simulink model "gg_plus_lc_platoon"  (R2019a)
settings: Solver=ode23t  StartTime=0.0  StopTime=70  FixedStep=0.1  MaxStep=0.01  RelTol=1e-3
InitFcn:
  | load vehStatesBus
libraries: simulink x120, powerlib_meascontrol x14, dspsigops x7, autolibshared x7
(part 2 of 7)

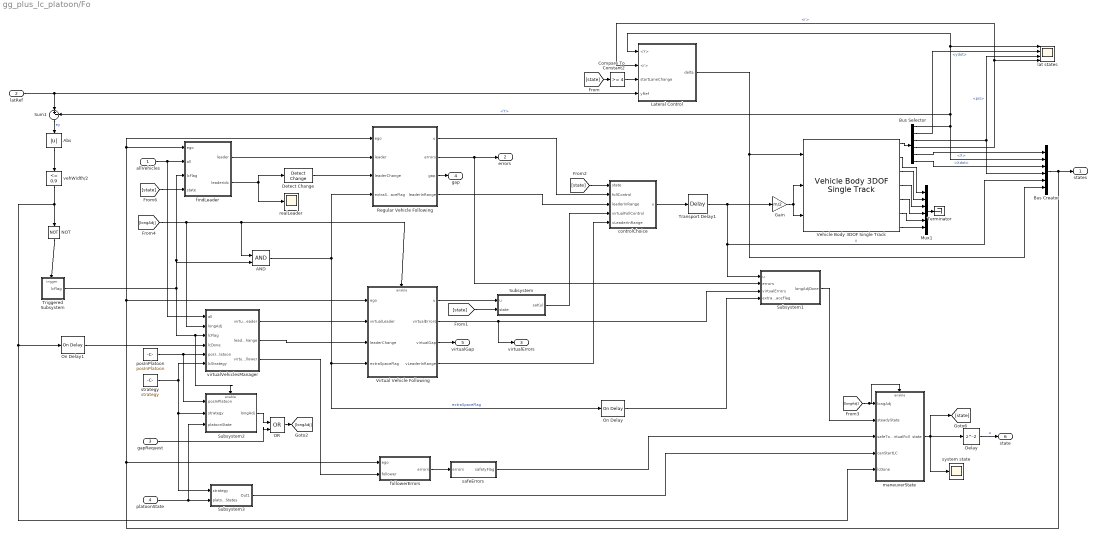
== system gg_plus_lc_platoon/Fo ==
  allVehicles : Inport
  latRef : Inport  Port=2
  gapRequest : Inport  Port=3
  platoonState : Inport  Port=4
  AND : Logic  IconShape=distinctive  AllPortsSameDT=off  OutDataTypeStr=boolean
  Abs : Abs
  Bus Creator : BusCreator  Inputs=6  OutDataTypeStr=Bus: vehStatesBus  NonVirtualBus=on
  Bus Selector : BusSelector  OutputSignals=InertFrm.Cg.Disp.Y,BdyFrm.Cg.Vel.ydot,InertFrm.Cg.Ang.psi,BdyFrm.Cg.AngVel.r,InertFrm.RearAxl.Disp.X,InertFrm.RearAxl.Vel.Xdot
  Compare To Constant2 : simulink/Logic and Bit Operations/Compare To Constant  relop=>=  const=4  OutDataTypeStr=boolean
  Delay : Delay
  Detect Change : simulink/Logic and Bit Operations/Detect Change  vinit=0  OutDataTypeStr=boolean
  Gain : Gain  Gain=m/2
  Lateral Control : Subsystem
  Mux1 : Mux  Inputs=6
  NOT : Logic  Operator=NOT  IconShape=distinctive  AllPortsSameDT=off  OutDataTypeStr=boolean
  OR : Logic  Operator=OR  IconShape=distinctive  AllPortsSameDT=off  OutDataTypeStr=boolean
  On Delay : powerlib_meascontrol/Logic/On Delay  DelayType=On delay  delay=1  ic=0  Ts=0
      settings: SourceProductName=Simscape Electrical
  On Delay1 : powerlib_meascontrol/Logic/On Delay  DelayType=On delay  delay=0.1  ic=0  Ts=0
      settings: SourceProductName=Simscape Electrical
  Regular Vehicle Following : Subsystem
  Subsystem : Subsystem
  Subsystem1 : Subsystem
  Subsystem2 : Subsystem
  Subsystem3 : Subsystem
  Sum1 : Sum  Inputs=|+-
  Terminator : Terminator
  Transport Delay1 : TransportDelay  DelayTime=0.01
  Triggered Subsystem : Subsystem  TreatAsAtomicUnit=on
  Vehicle Body 3DOF Single Track : autolibshared/Vehicle Body 3DOF Single Track  trackMode=Single (bicycle)  inputMode=External longitudinal forces  frontSteerMode=on  rearSteerMode=off  windMode=off  muMode=off  extFMode=off  extMMode=off  extXo=off  extpsio=off  extxdoto=off  extro=off  extYo=off  extTamb=off  extydoto=off  aMode=2  NF=2  NR=2  m=m  a=lf  b=lr  h=0.35  X_o=x0  xdot_o=vx0  CalphaMode=off  sigmaMode=on  d=0  w=[1.4,1.4]  Cy_f=12e3  Cy_r=11e3  sigma_f=.1  sigma_r=.1  alpha_f_brk=[-.1 .1]  Cy_f_data=[-9e3 9e3]  alpha_r_brk=[-.1 .1]  Cy_r_data=[-9e3 9e3]  Y_o=y0  ydot_o=0  Izz=4000  psi_o=0  r_o=0  Af=2  Cd=.3  Cl=.1  Cpm=.1  beta_w=[0:0.01:0.3]  Cs=[0:0.03:0.9]  Cym=[0:0.01:0.3]  Pabs=101325  Tair=273  g=9.81  mu=1  xdot_tol=.01  Fznom=5000  Fxtire_sat=7e4  Fytire_sat=7e4  longOff=0  latOff=0  vertOff=0  wrapAng=off
      settings: SourceProductName=Powertrain Blockset  SourceProductBaseCode=PW
  Virtual Vehicle Following : Subsystem  TreatAsAtomicUnit=on
  controlChoice : Subsystem
  findLeader : Subsystem
  followerErrors : Subsystem
  lat states : Scope  NumInputPorts=4
  maneuverState : Subsystem
  posInPlatoon : Constant  Value=posInPlatoon
  realLeader : Scope
  safeErrors : Subsystem
  strategy : Constant  Value=strategy
  system state : Scope
  vehWidth/2 : simulink/Logic and Bit Operations/Compare To Constant  relop=<=  const=0.9  OutDataTypeStr=boolean
  virtualVehiclesManager : Subsystem  TreatAsAtomicUnit=on
  states : Outport
  errors : Outport  Port=2
  virtualErrors : Outport  Port=3
  gap : Outport  Port=4
  virtualGap : Outport  Port=5
  state : Outport  Port=6
  wires:
  Triggered Subsystem/1(lcFlag) -> Subsystem2/Enable, virtualVehiclesManager/3(lcFlag), findLeader/3(lcFlag), AND/2
  Virtual Vehicle Following/4(vLeaderInRange) -> controlChoice/5(vLeaderInRange)
  [state] -> findLeader/4(state)
  Subsystem3/1(Out1) -> maneuverState/4(canStartLC)
  strategy/1 -> virtualVehiclesManager/6(lcStrategy), Subsystem3/1(strategy), Subsystem2/2(strategy)
  Delay/1 -> state/1  "u"
  Subsystem2/1(longAdj) -> OR/1
  platoonState/1 -> Subsystem2/3(platoonState), Subsystem3/2(platoonStates)
  [state] -> Compare To Constant2/1
  Virtual Vehicle Following/3(virtualGap) -> virtualGap/1
  maneuverState/1(state) -> Delay/1, [state], system state/1
  Lateral Control/1(delta) -> Bus Creator/6, Vehicle Body 3DOF Single Track/1
  Compare To Constant2/1 -> Lateral Control/3(startLaneChange)
  Regular Vehicle Following/2(errors) -> errors/1, Subsystem1/2(errors)
  Virtual Vehicle Following/1(u) -> Subsystem/1(u)
  Regular Vehicle Following/1(u) -> controlChoice/2(follControl)
  Regular Vehicle Following/3(gap) -> gap/1
  followerErrors/1(errors) -> safeErrors/1(errors)
  allVehicles/1 -> virtualVehiclesManager/1(all), findLeader/2(all)
  Abs/1 -> vehWidth/2/1
  AND/1 -> Regular Vehicle Following/4(extraSpaceFlag), On Delay/1, Virtual Vehicle Following/4(extraSpaceFlag)  "extraSpaceFlag"
  Bus Selector/6 -> Bus Creator/3  "<Xdot>"
  Bus Selector/5 -> Bus Creator/1  "<X>"
  Gain/1 -> Vehicle Body 3DOF Single Track/2, Vehicle Body 3DOF Single Track/3
  Vehicle Body 3DOF Single Track/1 -> Bus Selector/1
  Vehicle Body 3DOF Single Track/4 -> Mux1/3
  Vehicle Body 3DOF Single Track/3 -> Mux1/2
  Vehicle Body 3DOF Single Track/2 -> Mux1/1
  Vehicle Body 3DOF Single Track/5 -> Mux1/4
  Vehicle Body 3DOF Single Track/6 -> Mux1/5
  Vehicle Body 3DOF Single Track/7 -> Mux1/6
  Mux1/1 -> Terminator/1
  Bus Selector/1 -> Bus Creator/2, lat states/1, Lateral Control/1(<Y>), Sum1/2  "<Y>"
  Bus Selector/2 -> lat states/2  "<ydot>"
  Bus Selector/3 -> Bus Creator/4, lat states/3  "<psi>"
  Bus Selector/4 -> lat states/4, Lateral Control/2(<r>)  "<r>"
  latRef/1 -> Sum1/1, Lateral Control/4(yRef)
  Bus Creator/1 -> Regular Vehicle Following/1(ego), findLeader/1(ego), Virtual Vehicle Following/1(ego), followerErrors/1(ego), states/1
  Transport Delay1/1 -> Gain/1, Subsystem1/1(u), Bus Creator/5  "u"
  Sum1/1 -> Abs/1  "ey"
  Virtual Vehicle Following/2(virtualErrors) -> virtualErrors/1, Subsystem1/3(virtualErrors)
  Detect Change/1 -> Regular Vehicle Following/3(leaderChange)
  Subsystem/1(sat(u)) -> controlChoice/4(virtualFollControl)
  Regular Vehicle Following/4(leaderInRange) -> controlChoice/3(leaderInRange)
  findLeader/1(leader) -> Regular Vehicle Following/2(leader)
  findLeader/2(leaderIdx) -> Detect Change/1, realLeader/1
  On Delay/1 -> Subsystem1/4(extraSpaceFlag)
  NOT/1 -> Triggered Subsystem/Trigger
  [state] -> Subsystem/2(state)
  posInPlatoon/1 -> virtualVehiclesManager/5(posInPlatoon), Subsystem2/1(posInPlatoon)
  virtualVehiclesManager/1(virtualLeader) -> Virtual Vehicle Following/2(virtualLeader)
  virtualVehiclesManager/3(virtualFollower) -> followerErrors/2(follower)
  [longAdj] -> maneuverState/Enable, maneuverState/1(longAdj)
  Subsystem1/1(longAdjDone) -> maneuverState/2(steadyState)
  safeErrors/1(safetyFlag) -> maneuverState/3(safeToVirtualFoll)
  vehWidth/2/1 -> On Delay1/1, maneuverState/5(lcDone), NOT/1
  [state] -> controlChoice/1(state)
  controlChoice/1(u) -> Transport Delay1/1
  [longAdj] -> virtualVehiclesManager/2(longAdj), AND/1, Virtual Vehicle Following/Enable
  On Delay1/1 -> virtualVehiclesManager/4(lcDone)
  virtualVehiclesManager/2(leaderChange) -> Virtual Vehicle Following/3(leaderChange)
  OR/1 -> [longAdj]
  gapRequest/1 -> OR/2

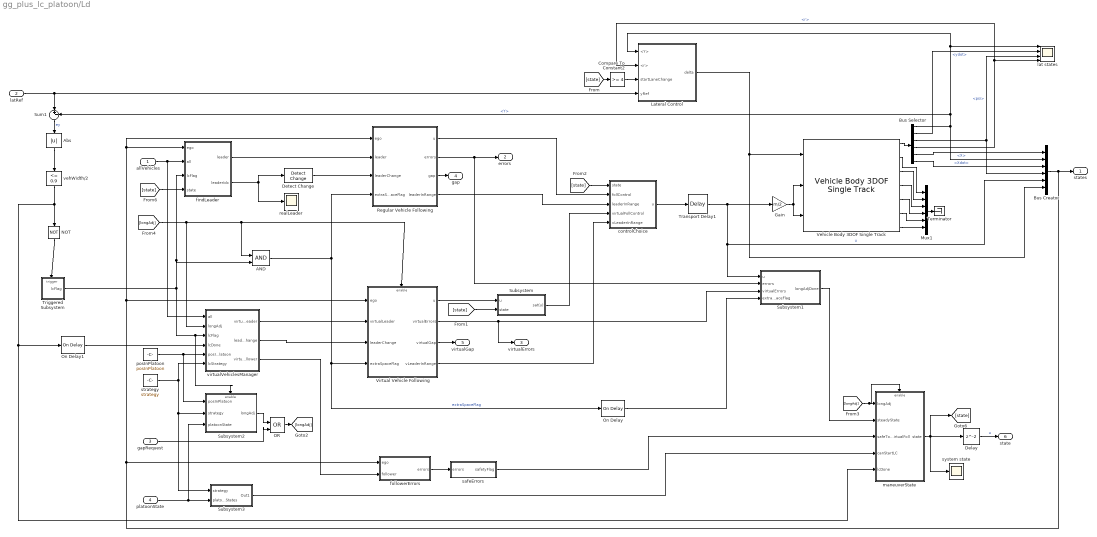
== system gg_plus_lc_platoon/Ld ==
  allVehicles : Inport
  latRef : Inport  Port=2
  gapRequest : Inport  Port=3
  platoonState : Inport  Port=4
  AND : Logic  IconShape=distinctive  AllPortsSameDT=off  OutDataTypeStr=boolean
  Abs : Abs
  Bus Creator : BusCreator  Inputs=6  OutDataTypeStr=Bus: vehStatesBus  NonVirtualBus=on
  Bus Selector : BusSelector  OutputSignals=InertFrm.Cg.Disp.Y,BdyFrm.Cg.Vel.ydot,InertFrm.Cg.Ang.psi,BdyFrm.Cg.AngVel.r,InertFrm.RearAxl.Disp.X,InertFrm.RearAxl.Vel.Xdot
  Compare To Constant2 : simulink/Logic and Bit Operations/Compare To Constant  relop=>=  const=4  OutDataTypeStr=boolean
  Delay : Delay
  Detect Change : simulink/Logic and Bit Operations/Detect Change  vinit=0  OutDataTypeStr=boolean
  Gain : Gain  Gain=m/2
  Lateral Control : Subsystem
  Mux1 : Mux  Inputs=6
  NOT : Logic  Operator=NOT  IconShape=distinctive  AllPortsSameDT=off  OutDataTypeStr=boolean
  OR : Logic  Operator=OR  IconShape=distinctive  AllPortsSameDT=off  OutDataTypeStr=boolean
  On Delay : powerlib_meascontrol/Logic/On Delay  DelayType=On delay  delay=1  ic=0  Ts=0
      settings: SourceProductName=Simscape Electrical
  On Delay1 : powerlib_meascontrol/Logic/On Delay  DelayType=On delay  delay=0.1  ic=0  Ts=0
      settings: SourceProductName=Simscape Electrical
  Regular Vehicle Following : Subsystem
  Subsystem : Subsystem
  Subsystem1 : Subsystem
  Subsystem2 : Subsystem
  Subsystem3 : Subsystem
  Sum1 : Sum  Inputs=|+-
  Terminator : Terminator
  Transport Delay1 : TransportDelay  DelayTime=0.01
  Triggered Subsystem : Subsystem  TreatAsAtomicUnit=on
  Vehicle Body 3DOF Single Track : autolibshared/Vehicle Body 3DOF Single Track  trackMode=Single (bicycle)  inputMode=External longitudinal forces  frontSteerMode=on  rearSteerMode=off  windMode=off  muMode=off  extFMode=off  extMMode=off  extXo=off  extpsio=off  extxdoto=off  extro=off  extYo=off  extTamb=off  extydoto=off  aMode=2  NF=2  NR=2  m=m  a=lf  b=lr  h=0.35  X_o=x0  xdot_o=vx0  CalphaMode=off  sigmaMode=on  d=0  w=[1.4,1.4]  Cy_f=12e3  Cy_r=11e3  sigma_f=.1  sigma_r=.1  alpha_f_brk=[-.1 .1]  Cy_f_data=[-9e3 9e3]  alpha_r_brk=[-.1 .1]  Cy_r_data=[-9e3 9e3]  Y_o=y0  ydot_o=0  Izz=4000  psi_o=0  r_o=0  Af=2  Cd=.3  Cl=.1  Cpm=.1  beta_w=[0:0.01:0.3]  Cs=[0:0.03:0.9]  Cym=[0:0.01:0.3]  Pabs=101325  Tair=273  g=9.81  mu=1  xdot_tol=.01  Fznom=5000  Fxtire_sat=7e4  Fytire_sat=7e4  longOff=0  latOff=0  vertOff=0  wrapAng=off
      settings: SourceProductName=Powertrain Blockset  SourceProductBaseCode=PW
  Virtual Vehicle Following : Subsystem  TreatAsAtomicUnit=on
  controlChoice : Subsystem
  findLeader : Subsystem
  followerErrors : Subsystem
  lat states : Scope  NumInputPorts=4
  maneuverState : Subsystem
  posInPlatoon : Constant  Value=posInPlatoon
  realLeader : Scope
  safeErrors : Subsystem
  strategy : Constant  Value=strategy
  system state : Scope
  vehWidth/2 : simulink/Logic and Bit Operations/Compare To Constant  relop=<=  const=0.9  OutDataTypeStr=boolean
  virtualVehiclesManager : Subsystem  TreatAsAtomicUnit=on
  states : Outport
  errors : Outport  Port=2
  virtualErrors : Outport  Port=3
  gap : Outport  Port=4
  virtualGap : Outport  Port=5
  state : Outport  Port=6
  wires:
  Triggered Subsystem/1(lcFlag) -> Subsystem2/Enable, virtualVehiclesManager/3(lcFlag), findLeader/3(lcFlag), AND/2
  Virtual Vehicle Following/4(vLeaderInRange) -> controlChoice/5(vLeaderInRange)
  [state] -> findLeader/4(state)
  Subsystem3/1(Out1) -> maneuverState/4(canStartLC)
  strategy/1 -> virtualVehiclesManager/6(lcStrategy), Subsystem3/1(strategy), Subsystem2/2(strategy)
  Delay/1 -> state/1  "u"
  Subsystem2/1(longAdj) -> OR/1
  platoonState/1 -> Subsystem2/3(platoonState), Subsystem3/2(platoonStates)
  [state] -> Compare To Constant2/1
  Virtual Vehicle Following/3(virtualGap) -> virtualGap/1
  maneuverState/1(state) -> Delay/1, [state], system state/1
  Lateral Control/1(delta) -> Bus Creator/6, Vehicle Body 3DOF Single Track/1
  Compare To Constant2/1 -> Lateral Control/3(startLaneChange)
  Regular Vehicle Following/2(errors) -> errors/1, Subsystem1/2(errors)
  Virtual Vehicle Following/1(u) -> Subsystem/1(u)
  Regular Vehicle Following/1(u) -> controlChoice/2(follControl)
  Regular Vehicle Following/3(gap) -> gap/1
  followerErrors/1(errors) -> safeErrors/1(errors)
  allVehicles/1 -> virtualVehiclesManager/1(all), findLeader/2(all)
  Abs/1 -> vehWidth/2/1
  AND/1 -> Regular Vehicle Following/4(extraSpaceFlag), On Delay/1, Virtual Vehicle Following/4(extraSpaceFlag)  "extraSpaceFlag"
  Bus Selector/6 -> Bus Creator/3  "<Xdot>"
  Bus Selector/5 -> Bus Creator/1  "<X>"
  Gain/1 -> Vehicle Body 3DOF Single Track/2, Vehicle Body 3DOF Single Track/3
  Vehicle Body 3DOF Single Track/1 -> Bus Selector/1
  Vehicle Body 3DOF Single Track/4 -> Mux1/3
  Vehicle Body 3DOF Single Track/3 -> Mux1/2
  Vehicle Body 3DOF Single Track/2 -> Mux1/1
  Vehicle Body 3DOF Single Track/5 -> Mux1/4
  Vehicle Body 3DOF Single Track/6 -> Mux1/5
  Vehicle Body 3DOF Single Track/7 -> Mux1/6
  Mux1/1 -> Terminator/1
  Bus Selector/1 -> Bus Creator/2, lat states/1, Lateral Control/1(<Y>), Sum1/2  "<Y>"
  Bus Selector/2 -> lat states/2  "<ydot>"
  Bus Selector/3 -> Bus Creator/4, lat states/3  "<psi>"
  Bus Selector/4 -> lat states/4, Lateral Control/2(<r>)  "<r>"
  latRef/1 -> Sum1/1, Lateral Control/4(yRef)
  Bus Creator/1 -> Regular Vehicle Following/1(ego), findLeader/1(ego), Virtual Vehicle Following/1(ego), followerErrors/1(ego), states/1
  Transport Delay1/1 -> Gain/1, Subsystem1/1(u), Bus Creator/5  "u"
  Sum1/1 -> Abs/1  "ey"
  Virtual Vehicle Following/2(virtualErrors) -> virtualErrors/1, Subsystem1/3(virtualErrors)
  Detect Change/1 -> Regular Vehicle Following/3(leaderChange)
  Subsystem/1(sat(u)) -> controlChoice/4(virtualFollControl)
  Regular Vehicle Following/4(leaderInRange) -> controlChoice/3(leaderInRange)
  findLeader/1(leader) -> Regular Vehicle Following/2(leader)
  findLeader/2(leaderIdx) -> Detect Change/1, realLeader/1
  On Delay/1 -> Subsystem1/4(extraSpaceFlag)
  NOT/1 -> Triggered Subsystem/Trigger
  [state] -> Subsystem/2(state)
  posInPlatoon/1 -> virtualVehiclesManager/5(posInPlatoon), Subsystem2/1(posInPlatoon)
  virtualVehiclesManager/1(virtualLeader) -> Virtual Vehicle Following/2(virtualLeader)
  virtualVehiclesManager/3(virtualFollower) -> followerErrors/2(follower)
  [longAdj] -> maneuverState/Enable, maneuverState/1(longAdj)
  Subsystem1/1(longAdjDone) -> maneuverState/2(steadyState)
  safeErrors/1(safetyFlag) -> maneuverState/3(safeToVirtualFoll)
  vehWidth/2/1 -> On Delay1/1, maneuverState/5(lcDone), NOT/1
  [state] -> controlChoice/1(state)
  controlChoice/1(u) -> Transport Delay1/1
  [longAdj] -> virtualVehiclesManager/2(longAdj), AND/1, Virtual Vehicle Following/Enable
  On Delay1/1 -> virtualVehiclesManager/4(lcDone)
  virtualVehiclesManager/2(leaderChange) -> Virtual Vehicle Following/3(leaderChange)
  OR/1 -> [longAdj]
  gapRequest/1 -> OR/2

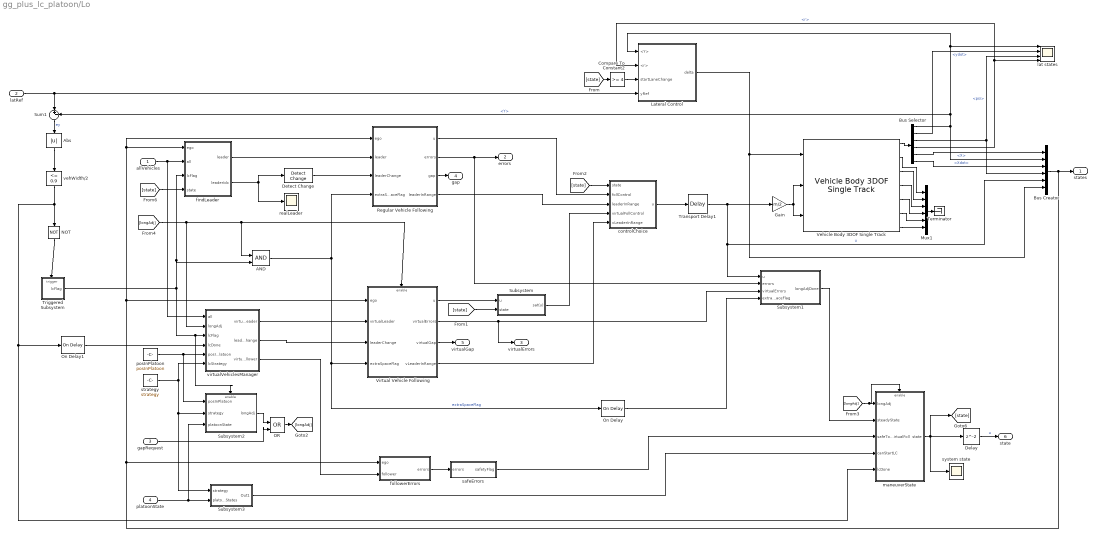
== system gg_plus_lc_platoon/Lo ==
  allVehicles : Inport
  latRef : Inport  Port=2
  gapRequest : Inport  Port=3
  platoonState : Inport  Port=4
  AND : Logic  IconShape=distinctive  AllPortsSameDT=off  OutDataTypeStr=boolean
  Abs : Abs
  Bus Creator : BusCreator  Inputs=6  OutDataTypeStr=Bus: vehStatesBus  NonVirtualBus=on
  Bus Selector : BusSelector  OutputSignals=InertFrm.Cg.Disp.Y,BdyFrm.Cg.Vel.ydot,InertFrm.Cg.Ang.psi,BdyFrm.Cg.AngVel.r,InertFrm.RearAxl.Disp.X,InertFrm.RearAxl.Vel.Xdot
  Compare To Constant2 : simulink/Logic and Bit Operations/Compare To Constant  relop=>=  const=4  OutDataTypeStr=boolean
  Delay : Delay
  Detect Change : simulink/Logic and Bit Operations/Detect Change  vinit=0  OutDataTypeStr=boolean
  Gain : Gain  Gain=m/2
  Lateral Control : Subsystem
  Mux1 : Mux  Inputs=6
  NOT : Logic  Operator=NOT  IconShape=distinctive  AllPortsSameDT=off  OutDataTypeStr=boolean
  OR : Logic  Operator=OR  IconShape=distinctive  AllPortsSameDT=off  OutDataTypeStr=boolean
  On Delay : powerlib_meascontrol/Logic/On Delay  DelayType=On delay  delay=1  ic=0  Ts=0
      settings: SourceProductName=Simscape Electrical
  On Delay1 : powerlib_meascontrol/Logic/On Delay  DelayType=On delay  delay=0.1  ic=0  Ts=0
      settings: SourceProductName=Simscape Electrical
  Regular Vehicle Following : Subsystem
  Subsystem : Subsystem
  Subsystem1 : Subsystem
  Subsystem2 : Subsystem
  Subsystem3 : Subsystem
  Sum1 : Sum  Inputs=|+-
  Terminator : Terminator
  Transport Delay1 : TransportDelay  DelayTime=0.01
  Triggered Subsystem : Subsystem  TreatAsAtomicUnit=on
  Vehicle Body 3DOF Single Track : autolibshared/Vehicle Body 3DOF Single Track  trackMode=Single (bicycle)  inputMode=External longitudinal forces  frontSteerMode=on  rearSteerMode=off  windMode=off  muMode=off  extFMode=off  extMMode=off  extXo=off  extpsio=off  extxdoto=off  extro=off  extYo=off  extTamb=off  extydoto=off  aMode=2  NF=2  NR=2  m=m  a=lf  b=lr  h=0.35  X_o=x0  xdot_o=vx0  CalphaMode=off  sigmaMode=on  d=0  w=[1.4,1.4]  Cy_f=12e3  Cy_r=11e3  sigma_f=.1  sigma_r=.1  alpha_f_brk=[-.1 .1]  Cy_f_data=[-9e3 9e3]  alpha_r_brk=[-.1 .1]  Cy_r_data=[-9e3 9e3]  Y_o=y0  ydot_o=0  Izz=4000  psi_o=0  r_o=0  Af=2  Cd=.3  Cl=.1  Cpm=.1  beta_w=[0:0.01:0.3]  Cs=[0:0.03:0.9]  Cym=[0:0.01:0.3]  Pabs=101325  Tair=273  g=9.81  mu=1  xdot_tol=.01  Fznom=5000  Fxtire_sat=7e4  Fytire_sat=7e4  longOff=0  latOff=0  vertOff=0  wrapAng=off
      settings: SourceProductName=Powertrain Blockset  SourceProductBaseCode=PW
  Virtual Vehicle Following : Subsystem  TreatAsAtomicUnit=on
  controlChoice : Subsystem
  findLeader : Subsystem
  followerErrors : Subsystem
  lat states : Scope  NumInputPorts=4
  maneuverState : Subsystem
  posInPlatoon : Constant  Value=posInPlatoon
  realLeader : Scope
  safeErrors : Subsystem
  strategy : Constant  Value=strategy
  system state : Scope
  vehWidth/2 : simulink/Logic and Bit Operations/Compare To Constant  relop=<=  const=0.9  OutDataTypeStr=boolean
  virtualVehiclesManager : Subsystem  TreatAsAtomicUnit=on
  states : Outport
  errors : Outport  Port=2
  virtualErrors : Outport  Port=3
  gap : Outport  Port=4
  virtualGap : Outport  Port=5
  state : Outport  Port=6
  wires:
  gapRequest/1 -> OR/2
  OR/1 -> [longAdj]
  virtualVehiclesManager/2(leaderChange) -> Virtual Vehicle Following/3(leaderChange)
  On Delay1/1 -> virtualVehiclesManager/4(lcDone)
  [longAdj] -> Virtual Vehicle Following/Enable, AND/1, virtualVehiclesManager/2(longAdj)
  controlChoice/1(u) -> Transport Delay1/1
  [state] -> controlChoice/1(state)
  vehWidth/2/1 -> NOT/1, maneuverState/5(lcDone), On Delay1/1
  safeErrors/1(safetyFlag) -> maneuverState/3(safeToVirtualFoll)
  Subsystem1/1(longAdjDone) -> maneuverState/2(steadyState)
  [longAdj] -> maneuverState/1(longAdj), maneuverState/Enable
  virtualVehiclesManager/3(virtualFollower) -> followerErrors/2(follower)
  virtualVehiclesManager/1(virtualLeader) -> Virtual Vehicle Following/2(virtualLeader)
  posInPlatoon/1 -> Subsystem2/1(posInPlatoon), virtualVehiclesManager/5(posInPlatoon)
  [state] -> Subsystem/2(state)
  NOT/1 -> Triggered Subsystem/Trigger
  On Delay/1 -> Subsystem1/4(extraSpaceFlag)
  findLeader/2(leaderIdx) -> realLeader/1, Detect Change/1
  findLeader/1(leader) -> Regular Vehicle Following/2(leader)
  Regular Vehicle Following/4(leaderInRange) -> controlChoice/3(leaderInRange)
  Subsystem/1(sat(u)) -> controlChoice/4(virtualFollControl)
  Detect Change/1 -> Regular Vehicle Following/3(leaderChange)
  Virtual Vehicle Following/2(virtualErrors) -> Subsystem1/3(virtualErrors), virtualErrors/1
  Sum1/1 -> Abs/1  "ey"
  Transport Delay1/1 -> Bus Creator/5, Subsystem1/1(u), Gain/1  "u"
  Bus Creator/1 -> states/1, followerErrors/1(ego), Virtual Vehicle Following/1(ego), findLeader/1(ego), Regular Vehicle Following/1(ego)
  latRef/1 -> Lateral Control/4(yRef), Sum1/1
  Bus Selector/4 -> Lateral Control/2(<r>), lat states/4  "<r>"
  Bus Selector/3 -> lat states/3, Bus Creator/4  "<psi>"
  Bus Selector/2 -> lat states/2  "<ydot>"
  Bus Selector/1 -> Sum1/2, Lateral Control/1(<Y>), lat states/1, Bus Creator/2  "<Y>"
  Mux1/1 -> Terminator/1
  Vehicle Body 3DOF Single Track/7 -> Mux1/6
  Vehicle Body 3DOF Single Track/6 -> Mux1/5
  Vehicle Body 3DOF Single Track/5 -> Mux1/4
  Vehicle Body 3DOF Single Track/2 -> Mux1/1
  Vehicle Body 3DOF Single Track/3 -> Mux1/2
  Vehicle Body 3DOF Single Track/4 -> Mux1/3
  Vehicle Body 3DOF Single Track/1 -> Bus Selector/1
  Gain/1 -> Vehicle Body 3DOF Single Track/3, Vehicle Body 3DOF Single Track/2
  Bus Selector/5 -> Bus Creator/1  "<X>"
  Bus Selector/6 -> Bus Creator/3  "<Xdot>"
  AND/1 -> Virtual Vehicle Following/4(extraSpaceFlag), On Delay/1, Regular Vehicle Following/4(extraSpaceFlag)  "extraSpaceFlag"
  Abs/1 -> vehWidth/2/1
  allVehicles/1 -> findLeader/2(all), virtualVehiclesManager/1(all)
  followerErrors/1(errors) -> safeErrors/1(errors)
  Regular Vehicle Following/3(gap) -> gap/1
  Regular Vehicle Following/1(u) -> controlChoice/2(follControl)
  Virtual Vehicle Following/1(u) -> Subsystem/1(u)
  Regular Vehicle Following/2(errors) -> Subsystem1/2(errors), errors/1
  Compare To Constant2/1 -> Lateral Control/3(startLaneChange)
  Lateral Control/1(delta) -> Vehicle Body 3DOF Single Track/1, Bus Creator/6
  maneuverState/1(state) -> system state/1, [state], Delay/1
  Virtual Vehicle Following/3(virtualGap) -> virtualGap/1
  [state] -> Compare To Constant2/1
  platoonState/1 -> Subsystem3/2(platoonStates), Subsystem2/3(platoonState)
  Subsystem2/1(longAdj) -> OR/1
  Delay/1 -> state/1  "u"
  strategy/1 -> Subsystem2/2(strategy), Subsystem3/1(strategy), virtualVehiclesManager/6(lcStrategy)
  Subsystem3/1(Out1) -> maneuverState/4(canStartLC)
  [state] -> findLeader/4(state)
  Virtual Vehicle Following/4(vLeaderInRange) -> controlChoice/5(vLeaderInRange)
  Triggered Subsystem/1(lcFlag) -> AND/2, findLeader/3(lcFlag), virtualVehiclesManager/3(lcFlag), Subsystem2/Enable

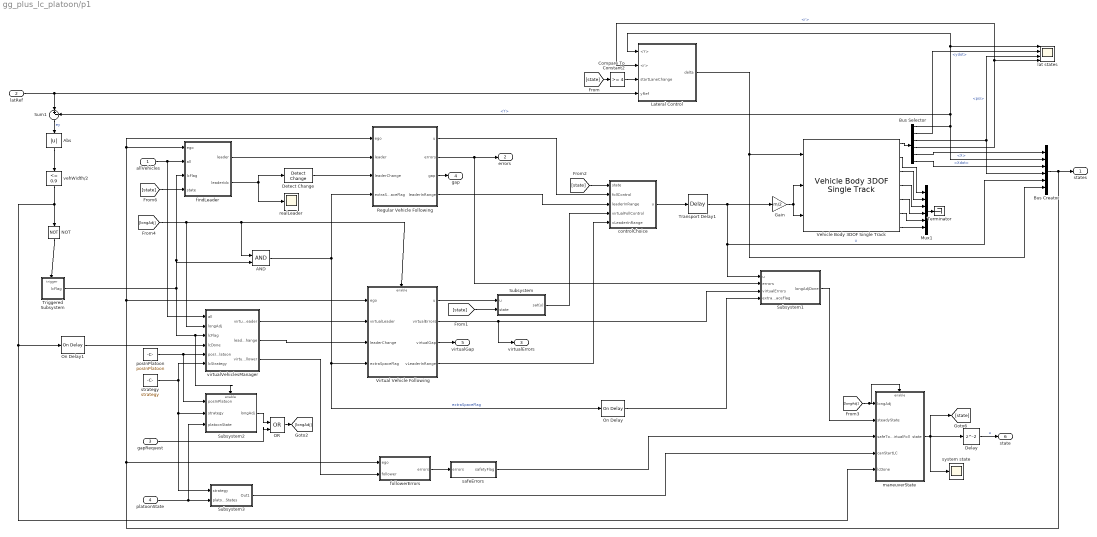
== system gg_plus_lc_platoon/p1 ==
  allVehicles : Inport
  latRef : Inport  Port=2
  gapRequest : Inport  Port=3
  platoonState : Inport  Port=4
  AND : Logic  IconShape=distinctive  AllPortsSameDT=off  OutDataTypeStr=boolean
  Abs : Abs
  Bus Creator : BusCreator  Inputs=6  OutDataTypeStr=Bus: vehStatesBus  NonVirtualBus=on
  Bus Selector : BusSelector  OutputSignals=InertFrm.Cg.Disp.Y,BdyFrm.Cg.Vel.ydot,InertFrm.Cg.Ang.psi,BdyFrm.Cg.AngVel.r,InertFrm.RearAxl.Disp.X,InertFrm.RearAxl.Vel.Xdot
  Compare To Constant2 : simulink/Logic and Bit Operations/Compare To Constant  relop=>=  const=4  OutDataTypeStr=boolean
  Delay : Delay
  Detect Change : simulink/Logic and Bit Operations/Detect Change  vinit=0  OutDataTypeStr=boolean
  Gain : Gain  Gain=m/2
  Lateral Control : Subsystem
  Mux1 : Mux  Inputs=6
  NOT : Logic  Operator=NOT  IconShape=distinctive  AllPortsSameDT=off  OutDataTypeStr=boolean
  OR : Logic  Operator=OR  IconShape=distinctive  AllPortsSameDT=off  OutDataTypeStr=boolean
  On Delay : powerlib_meascontrol/Logic/On Delay  DelayType=On delay  delay=1  ic=0  Ts=0
      settings: SourceProductName=Simscape Electrical
  On Delay1 : powerlib_meascontrol/Logic/On Delay  DelayType=On delay  delay=0.1  ic=0  Ts=0
      settings: SourceProductName=Simscape Electrical
  Regular Vehicle Following : Subsystem
  Subsystem : Subsystem
  Subsystem1 : Subsystem
  Subsystem2 : Subsystem
  Subsystem3 : Subsystem
  Sum1 : Sum  Inputs=|+-
  Terminator : Terminator
  Transport Delay1 : TransportDelay  DelayTime=0.01
  Triggered Subsystem : Subsystem  TreatAsAtomicUnit=on
  Vehicle Body 3DOF Single Track : autolibshared/Vehicle Body 3DOF Single Track  trackMode=Single (bicycle)  inputMode=External longitudinal forces  frontSteerMode=on  rearSteerMode=off  windMode=off  muMode=off  extFMode=off  extMMode=off  extXo=off  extpsio=off  extxdoto=off  extro=off  extYo=off  extTamb=off  extydoto=off  aMode=2  NF=2  NR=2  m=m  a=lf  b=lr  h=0.35  X_o=x0  xdot_o=vx0  CalphaMode=off  sigmaMode=on  d=0  w=[1.4,1.4]  Cy_f=12e3  Cy_r=11e3  sigma_f=.1  sigma_r=.1  alpha_f_brk=[-.1 .1]  Cy_f_data=[-9e3 9e3]  alpha_r_brk=[-.1 .1]  Cy_r_data=[-9e3 9e3]  Y_o=y0  ydot_o=0  Izz=4000  psi_o=0  r_o=0  Af=2  Cd=.3  Cl=.1  Cpm=.1  beta_w=[0:0.01:0.3]  Cs=[0:0.03:0.9]  Cym=[0:0.01:0.3]  Pabs=101325  Tair=273  g=9.81  mu=1  xdot_tol=.01  Fznom=5000  Fxtire_sat=7e4  Fytire_sat=7e4  longOff=0  latOff=0  vertOff=0  wrapAng=off
      settings: SourceProductName=Powertrain Blockset  SourceProductBaseCode=PW
  Virtual Vehicle Following : Subsystem  TreatAsAtomicUnit=on
  controlChoice : Subsystem
  findLeader : Subsystem
  followerErrors : Subsystem
  lat states : Scope  NumInputPorts=4
  maneuverState : Subsystem
  posInPlatoon : Constant  Value=posInPlatoon
  realLeader : Scope
  safeErrors : Subsystem
  strategy : Constant  Value=strategy
  system state : Scope
  vehWidth/2 : simulink/Logic and Bit Operations/Compare To Constant  relop=<=  const=0.9  OutDataTypeStr=boolean
  virtualVehiclesManager : Subsystem  TreatAsAtomicUnit=on
  states : Outport
  errors : Outport  Port=2
  virtualErrors : Outport  Port=3
  gap : Outport  Port=4
  virtualGap : Outport  Port=5
  state : Outport  Port=6
  wires:
  Triggered Subsystem/1(lcFlag) -> Subsystem2/Enable, virtualVehiclesManager/3(lcFlag), findLeader/3(lcFlag), AND/2
  Virtual Vehicle Following/4(vLeaderInRange) -> controlChoice/5(vLeaderInRange)
  [state] -> findLeader/4(state)
  Subsystem3/1(Out1) -> maneuverState/4(canStartLC)
  strategy/1 -> virtualVehiclesManager/6(lcStrategy), Subsystem3/1(strategy), Subsystem2/2(strategy)
  Delay/1 -> state/1  "u"
  Subsystem2/1(longAdj) -> OR/1
  platoonState/1 -> Subsystem2/3(platoonState), Subsystem3/2(platoonStates)
  [state] -> Compare To Constant2/1
  Virtual Vehicle Following/3(virtualGap) -> virtualGap/1
  maneuverState/1(state) -> Delay/1, [state], system state/1
  Lateral Control/1(delta) -> Bus Creator/6, Vehicle Body 3DOF Single Track/1
  Compare To Constant2/1 -> Lateral Control/3(startLaneChange)
  Regular Vehicle Following/2(errors) -> errors/1, Subsystem1/2(errors)
  Virtual Vehicle Following/1(u) -> Subsystem/1(u)
  Regular Vehicle Following/1(u) -> controlChoice/2(follControl)
  Regular Vehicle Following/3(gap) -> gap/1
  followerErrors/1(errors) -> safeErrors/1(errors)
  allVehicles/1 -> virtualVehiclesManager/1(all), findLeader/2(all)
  Abs/1 -> vehWidth/2/1
  AND/1 -> Regular Vehicle Following/4(extraSpaceFlag), On Delay/1, Virtual Vehicle Following/4(extraSpaceFlag)  "extraSpaceFlag"
  Bus Selector/6 -> Bus Creator/3  "<Xdot>"
  Bus Selector/5 -> Bus Creator/1  "<X>"
  Gain/1 -> Vehicle Body 3DOF Single Track/2, Vehicle Body 3DOF Single Track/3
  Vehicle Body 3DOF Single Track/1 -> Bus Selector/1
  Vehicle Body 3DOF Single Track/4 -> Mux1/3
  Vehicle Body 3DOF Single Track/3 -> Mux1/2
  Vehicle Body 3DOF Single Track/2 -> Mux1/1
  Vehicle Body 3DOF Single Track/5 -> Mux1/4
  Vehicle Body 3DOF Single Track/6 -> Mux1/5
  Vehicle Body 3DOF Single Track/7 -> Mux1/6
  Mux1/1 -> Terminator/1
  Bus Selector/1 -> Bus Creator/2, lat states/1, Lateral Control/1(<Y>), Sum1/2  "<Y>"
  Bus Selector/2 -> lat states/2  "<ydot>"
  Bus Selector/3 -> Bus Creator/4, lat states/3  "<psi>"
  Bus Selector/4 -> lat states/4, Lateral Control/2(<r>)  "<r>"
  latRef/1 -> Sum1/1, Lateral Control/4(yRef)
  Bus Creator/1 -> Regular Vehicle Following/1(ego), findLeader/1(ego), Virtual Vehicle Following/1(ego), followerErrors/1(ego), states/1
  Transport Delay1/1 -> Gain/1, Subsystem1/1(u), Bus Creator/5  "u"
  Sum1/1 -> Abs/1  "ey"
  Virtual Vehicle Following/2(virtualErrors) -> virtualErrors/1, Subsystem1/3(virtualErrors)
  Detect Change/1 -> Regular Vehicle Following/3(leaderChange)
  Subsystem/1(sat(u)) -> controlChoice/4(virtualFollControl)
  Regular Vehicle Following/4(leaderInRange) -> controlChoice/3(leaderInRange)
  findLeader/1(leader) -> Regular Vehicle Following/2(leader)
  findLeader/2(leaderIdx) -> Detect Change/1, realLeader/1
  On Delay/1 -> Subsystem1/4(extraSpaceFlag)
  NOT/1 -> Triggered Subsystem/Trigger
  [state] -> Subsystem/2(state)
  posInPlatoon/1 -> virtualVehiclesManager/5(posInPlatoon), Subsystem2/1(posInPlatoon)
  virtualVehiclesManager/1(virtualLeader) -> Virtual Vehicle Following/2(virtualLeader)
  virtualVehiclesManager/3(virtualFollower) -> followerErrors/2(follower)
  [longAdj] -> maneuverState/Enable, maneuverState/1(longAdj)
  Subsystem1/1(longAdjDone) -> maneuverState/2(steadyState)
  safeErrors/1(safetyFlag) -> maneuverState/3(safeToVirtualFoll)
  vehWidth/2/1 -> On Delay1/1, maneuverState/5(lcDone), NOT/1
  [state] -> controlChoice/1(state)
  controlChoice/1(u) -> Transport Delay1/1
  [longAdj] -> virtualVehiclesManager/2(longAdj), AND/1, Virtual Vehicle Following/Enable
  On Delay1/1 -> virtualVehiclesManager/4(lcDone)
  virtualVehiclesManager/2(leaderChange) -> Virtual Vehicle Following/3(leaderChange)
  OR/1 -> [longAdj]
  gapRequest/1 -> OR/2

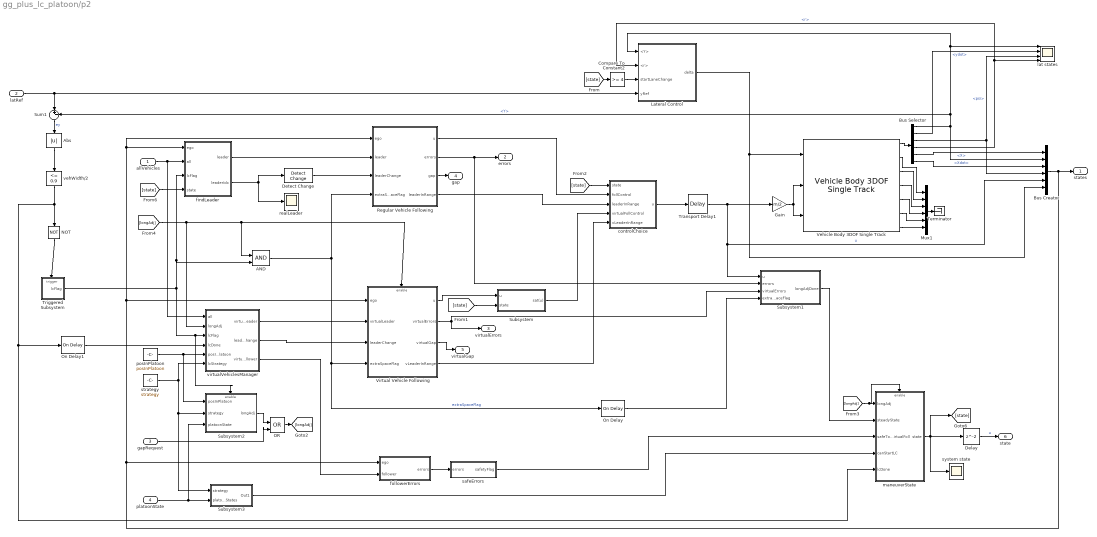
== system gg_plus_lc_platoon/p2 ==
  allVehicles : Inport
  latRef : Inport  Port=2
  gapRequest : Inport  Port=3
  platoonState : Inport  Port=4
  AND : Logic  IconShape=distinctive  AllPortsSameDT=off  OutDataTypeStr=boolean
  Abs : Abs
  Bus Creator : BusCreator  Inputs=6  OutDataTypeStr=Bus: vehStatesBus  NonVirtualBus=on
  Bus Selector : BusSelector  OutputSignals=InertFrm.Cg.Disp.Y,BdyFrm.Cg.Vel.ydot,InertFrm.Cg.Ang.psi,BdyFrm.Cg.AngVel.r,InertFrm.RearAxl.Disp.X,InertFrm.RearAxl.Vel.Xdot
  Compare To Constant2 : simulink/Logic and Bit Operations/Compare To Constant  relop=>=  const=4  OutDataTypeStr=boolean
  Delay : Delay
  Detect Change : simulink/Logic and Bit Operations/Detect Change  vinit=0  OutDataTypeStr=boolean
  Gain : Gain  Gain=m/2
  Lateral Control : Subsystem
  Mux1 : Mux  Inputs=6
  NOT : Logic  Operator=NOT  IconShape=distinctive  AllPortsSameDT=off  OutDataTypeStr=boolean
  OR : Logic  Operator=OR  IconShape=distinctive  AllPortsSameDT=off  OutDataTypeStr=boolean
  On Delay : powerlib_meascontrol/Logic/On Delay  DelayType=On delay  delay=1  ic=0  Ts=0
      settings: SourceProductName=Simscape Electrical
  On Delay1 : powerlib_meascontrol/Logic/On Delay  DelayType=On delay  delay=0.1  ic=0  Ts=0
      settings: SourceProductName=Simscape Electrical
  Regular Vehicle Following : Subsystem
  Subsystem : Subsystem
  Subsystem1 : Subsystem
  Subsystem2 : Subsystem
  Subsystem3 : Subsystem
  Sum1 : Sum  Inputs=|+-
  Terminator : Terminator
  Transport Delay1 : TransportDelay  DelayTime=0.01
  Triggered Subsystem : Subsystem  TreatAsAtomicUnit=on
  Vehicle Body 3DOF Single Track : autolibshared/Vehicle Body 3DOF Single Track  trackMode=Single (bicycle)  inputMode=External longitudinal forces  frontSteerMode=on  rearSteerMode=off  windMode=off  muMode=off  extFMode=off  extMMode=off  extXo=off  extpsio=off  extxdoto=off  extro=off  extYo=off  extTamb=off  extydoto=off  aMode=2  NF=2  NR=2  m=m  a=lf  b=lr  h=0.35  X_o=x0  xdot_o=vx0  CalphaMode=off  sigmaMode=on  d=0  w=[1.4,1.4]  Cy_f=12e3  Cy_r=11e3  sigma_f=.1  sigma_r=.1  alpha_f_brk=[-.1 .1]  Cy_f_data=[-9e3 9e3]  alpha_r_brk=[-.1 .1]  Cy_r_data=[-9e3 9e3]  Y_o=y0  ydot_o=0  Izz=4000  psi_o=0  r_o=0  Af=2  Cd=.3  Cl=.1  Cpm=.1  beta_w=[0:0.01:0.3]  Cs=[0:0.03:0.9]  Cym=[0:0.01:0.3]  Pabs=101325  Tair=273  g=9.81  mu=1  xdot_tol=.01  Fznom=5000  Fxtire_sat=7e4  Fytire_sat=7e4  longOff=0  latOff=0  vertOff=0  wrapAng=off
      settings: SourceProductName=Powertrain Blockset  SourceProductBaseCode=PW
  Virtual Vehicle Following : Subsystem  TreatAsAtomicUnit=on
  controlChoice : Subsystem
  findLeader : Subsystem
  followerErrors : Subsystem
  lat states : Scope  NumInputPorts=4
  maneuverState : Subsystem
  posInPlatoon : Constant  Value=posInPlatoon
  realLeader : Scope
  safeErrors : Subsystem
  strategy : Constant  Value=strategy
  system state : Scope
  vehWidth/2 : simulink/Logic and Bit Operations/Compare To Constant  relop=<=  const=0.9  OutDataTypeStr=boolean
  virtualVehiclesManager : Subsystem  TreatAsAtomicUnit=on
  states : Outport
  errors : Outport  Port=2
  virtualErrors : Outport  Port=3
  gap : Outport  Port=4
  virtualGap : Outport  Port=5
  state : Outport  Port=6
  wires:
  gapRequest/1 -> OR/2
  OR/1 -> [longAdj]
  virtualVehiclesManager/2(leaderChange) -> Virtual Vehicle Following/3(leaderChange)
  On Delay1/1 -> virtualVehiclesManager/4(lcDone)
  [longAdj] -> Virtual Vehicle Following/Enable, AND/1, virtualVehiclesManager/2(longAdj)
  controlChoice/1(u) -> Transport Delay1/1
  [state] -> controlChoice/1(state)
  vehWidth/2/1 -> NOT/1, maneuverState/5(lcDone), On Delay1/1
  safeErrors/1(safetyFlag) -> maneuverState/3(safeToVirtualFoll)
  Subsystem1/1(longAdjDone) -> maneuverState/2(steadyState)
  [longAdj] -> maneuverState/1(longAdj), maneuverState/Enable
  virtualVehiclesManager/3(virtualFollower) -> followerErrors/2(follower)
  virtualVehiclesManager/1(virtualLeader) -> Virtual Vehicle Following/2(virtualLeader)
  posInPlatoon/1 -> Subsystem2/1(posInPlatoon), virtualVehiclesManager/5(posInPlatoon)
  [state] -> Subsystem/2(state)
  NOT/1 -> Triggered Subsystem/Trigger
  On Delay/1 -> Subsystem1/4(extraSpaceFlag)
  findLeader/2(leaderIdx) -> realLeader/1, Detect Change/1
  findLeader/1(leader) -> Regular Vehicle Following/2(leader)
  Regular Vehicle Following/4(leaderInRange) -> controlChoice/3(leaderInRange)
  Subsystem/1(sat(u)) -> controlChoice/4(virtualFollControl)
  Detect Change/1 -> Regular Vehicle Following/3(leaderChange)
  Virtual Vehicle Following/2(virtualErrors) -> Subsystem1/3(virtualErrors), virtualErrors/1
  Sum1/1 -> Abs/1  "ey"
  Transport Delay1/1 -> Bus Creator/5, Subsystem1/1(u), Gain/1  "u"
  Bus Creator/1 -> states/1, followerErrors/1(ego), Virtual Vehicle Following/1(ego), findLeader/1(ego), Regular Vehicle Following/1(ego)
  latRef/1 -> Lateral Control/4(yRef), Sum1/1
  Bus Selector/4 -> Lateral Control/2(<r>), lat states/4  "<r>"
  Bus Selector/3 -> lat states/3, Bus Creator/4  "<psi>"
  Bus Selector/2 -> lat states/2  "<ydot>"
  Bus Selector/1 -> Sum1/2, Lateral Control/1(<Y>), lat states/1, Bus Creator/2  "<Y>"
  Mux1/1 -> Terminator/1
  Vehicle Body 3DOF Single Track/7 -> Mux1/6
  Vehicle Body 3DOF Single Track/6 -> Mux1/5
  Vehicle Body 3DOF Single Track/5 -> Mux1/4
  Vehicle Body 3DOF Single Track/2 -> Mux1/1
  Vehicle Body 3DOF Single Track/3 -> Mux1/2
  Vehicle Body 3DOF Single Track/4 -> Mux1/3
  Vehicle Body 3DOF Single Track/1 -> Bus Selector/1
  Gain/1 -> Vehicle Body 3DOF Single Track/3, Vehicle Body 3DOF Single Track/2
  Bus Selector/5 -> Bus Creator/1  "<X>"
  Bus Selector/6 -> Bus Creator/3  "<Xdot>"
  AND/1 -> Virtual Vehicle Following/4(extraSpaceFlag), On Delay/1, Regular Vehicle Following/4(extraSpaceFlag)  "extraSpaceFlag"
  Abs/1 -> vehWidth/2/1
  allVehicles/1 -> findLeader/2(all), virtualVehiclesManager/1(all)
  followerErrors/1(errors) -> safeErrors/1(errors)
  Regular Vehicle Following/3(gap) -> gap/1
  Regular Vehicle Following/1(u) -> controlChoice/2(follControl)
  Virtual Vehicle Following/1(u) -> Subsystem/1(u)
  Regular Vehicle Following/2(errors) -> Subsystem1/2(errors), errors/1
  Compare To Constant2/1 -> Lateral Control/3(startLaneChange)
  Lateral Control/1(delta) -> Vehicle Body 3DOF Single Track/1, Bus Creator/6
  maneuverState/1(state) -> system state/1, [state], Delay/1
  Virtual Vehicle Following/3(virtualGap) -> virtualGap/1
  [state] -> Compare To Constant2/1
  platoonState/1 -> Subsystem3/2(platoonStates), Subsystem2/3(platoonState)
  Subsystem2/1(longAdj) -> OR/1
  Delay/1 -> state/1  "u"
  strategy/1 -> Subsystem2/2(strategy), Subsystem3/1(strategy), virtualVehiclesManager/6(lcStrategy)
  Subsystem3/1(Out1) -> maneuverState/4(canStartLC)
  [state] -> findLeader/4(state)
  Virtual Vehicle Following/4(vLeaderInRange) -> controlChoice/5(vLeaderInRange)
  Triggered Subsystem/1(lcFlag) -> AND/2, findLeader/3(lcFlag), virtualVehiclesManager/3(lcFlag), Subsystem2/Enable

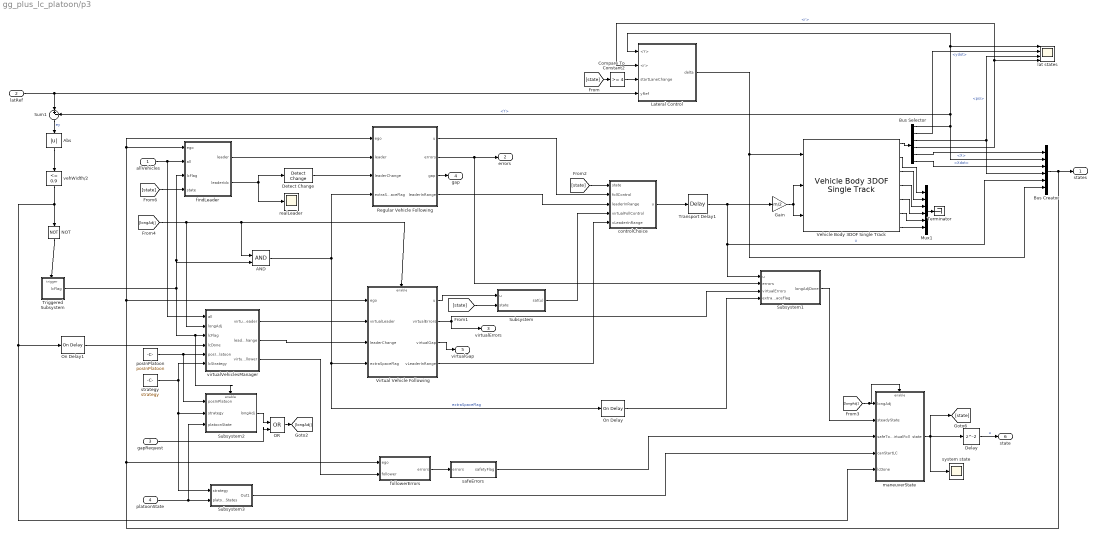
== system gg_plus_lc_platoon/p3 ==
  allVehicles : Inport
  latRef : Inport  Port=2
  gapRequest : Inport  Port=3
  platoonState : Inport  Port=4
  AND : Logic  IconShape=distinctive  AllPortsSameDT=off  OutDataTypeStr=boolean
  Abs : Abs
  Bus Creator : BusCreator  Inputs=6  OutDataTypeStr=Bus: vehStatesBus  NonVirtualBus=on
  Bus Selector : BusSelector  OutputSignals=InertFrm.Cg.Disp.Y,BdyFrm.Cg.Vel.ydot,InertFrm.Cg.Ang.psi,BdyFrm.Cg.AngVel.r,InertFrm.RearAxl.Disp.X,InertFrm.RearAxl.Vel.Xdot
  Compare To Constant2 : simulink/Logic and Bit Operations/Compare To Constant  relop=>=  const=4  OutDataTypeStr=boolean
  Delay : Delay
  Detect Change : simulink/Logic and Bit Operations/Detect Change  vinit=0  OutDataTypeStr=boolean
  Gain : Gain  Gain=m/2
  Lateral Control : Subsystem
  Mux1 : Mux  Inputs=6
  NOT : Logic  Operator=NOT  IconShape=distinctive  AllPortsSameDT=off  OutDataTypeStr=boolean
  OR : Logic  Operator=OR  IconShape=distinctive  AllPortsSameDT=off  OutDataTypeStr=boolean
  On Delay : powerlib_meascontrol/Logic/On Delay  DelayType=On delay  delay=1  ic=0  Ts=0
      settings: SourceProductName=Simscape Electrical
  On Delay1 : powerlib_meascontrol/Logic/On Delay  DelayType=On delay  delay=0.1  ic=0  Ts=0
      settings: SourceProductName=Simscape Electrical
  Regular Vehicle Following : Subsystem
  Subsystem : Subsystem
  Subsystem1 : Subsystem
  Subsystem2 : Subsystem
  Subsystem3 : Subsystem
  Sum1 : Sum  Inputs=|+-
  Terminator : Terminator
  Transport Delay1 : TransportDelay  DelayTime=0.01
  Triggered Subsystem : Subsystem  TreatAsAtomicUnit=on
  Vehicle Body 3DOF Single Track : autolibshared/Vehicle Body 3DOF Single Track  trackMode=Single (bicycle)  inputMode=External longitudinal forces  frontSteerMode=on  rearSteerMode=off  windMode=off  muMode=off  extFMode=off  extMMode=off  extXo=off  extpsio=off  extxdoto=off  extro=off  extYo=off  extTamb=off  extydoto=off  aMode=2  NF=2  NR=2  m=m  a=lf  b=lr  h=0.35  X_o=x0  xdot_o=vx0  CalphaMode=off  sigmaMode=on  d=0  w=[1.4,1.4]  Cy_f=12e3  Cy_r=11e3  sigma_f=.1  sigma_r=.1  alpha_f_brk=[-.1 .1]  Cy_f_data=[-9e3 9e3]  alpha_r_brk=[-.1 .1]  Cy_r_data=[-9e3 9e3]  Y_o=y0  ydot_o=0  Izz=4000  psi_o=0  r_o=0  Af=2  Cd=.3  Cl=.1  Cpm=.1  beta_w=[0:0.01:0.3]  Cs=[0:0.03:0.9]  Cym=[0:0.01:0.3]  Pabs=101325  Tair=273  g=9.81  mu=1  xdot_tol=.01  Fznom=5000  Fxtire_sat=7e4  Fytire_sat=7e4  longOff=0  latOff=0  vertOff=0  wrapAng=off
      settings: SourceProductName=Powertrain Blockset  SourceProductBaseCode=PW
  Virtual Vehicle Following : Subsystem  TreatAsAtomicUnit=on
  controlChoice : Subsystem
  findLeader : Subsystem
  followerErrors : Subsystem
  lat states : Scope  NumInputPorts=4
  maneuverState : Subsystem
  posInPlatoon : Constant  Value=posInPlatoon
  realLeader : Scope
  safeErrors : Subsystem
  strategy : Constant  Value=strategy
  system state : Scope
  vehWidth/2 : simulink/Logic and Bit Operations/Compare To Constant  relop=<=  const=0.9  OutDataTypeStr=boolean
  virtualVehiclesManager : Subsystem  TreatAsAtomicUnit=on
  states : Outport
  errors : Outport  Port=2
  virtualErrors : Outport  Port=3
  gap : Outport  Port=4
  virtualGap : Outport  Port=5
  state : Outport  Port=6
  wires:
  gapRequest/1 -> OR/2
  OR/1 -> [longAdj]
  virtualVehiclesManager/2(leaderChange) -> Virtual Vehicle Following/3(leaderChange)
  On Delay1/1 -> virtualVehiclesManager/4(lcDone)
  [longAdj] -> Virtual Vehicle Following/Enable, AND/1, virtualVehiclesManager/2(longAdj)
  controlChoice/1(u) -> Transport Delay1/1
  [state] -> controlChoice/1(state)
  vehWidth/2/1 -> NOT/1, maneuverState/5(lcDone), On Delay1/1
  safeErrors/1(safetyFlag) -> maneuverState/3(safeToVirtualFoll)
  Subsystem1/1(longAdjDone) -> maneuverState/2(steadyState)
  [longAdj] -> maneuverState/1(longAdj), maneuverState/Enable
  virtualVehiclesManager/3(virtualFollower) -> followerErrors/2(follower)
  virtualVehiclesManager/1(virtualLeader) -> Virtual Vehicle Following/2(virtualLeader)
  posInPlatoon/1 -> Subsystem2/1(posInPlatoon), virtualVehiclesManager/5(posInPlatoon)
  [state] -> Subsystem/2(state)
  NOT/1 -> Triggered Subsystem/Trigger
  On Delay/1 -> Subsystem1/4(extraSpaceFlag)
  findLeader/2(leaderIdx) -> realLeader/1, Detect Change/1
  findLeader/1(leader) -> Regular Vehicle Following/2(leader)
  Regular Vehicle Following/4(leaderInRange) -> controlChoice/3(leaderInRange)
  Subsystem/1(sat(u)) -> controlChoice/4(virtualFollControl)
  Detect Change/1 -> Regular Vehicle Following/3(leaderChange)
  Virtual Vehicle Following/2(virtualErrors) -> Subsystem1/3(virtualErrors), virtualErrors/1
  Sum1/1 -> Abs/1  "ey"
  Transport Delay1/1 -> Bus Creator/5, Subsystem1/1(u), Gain/1  "u"
  Bus Creator/1 -> states/1, followerErrors/1(ego), Virtual Vehicle Following/1(ego), findLeader/1(ego), Regular Vehicle Following/1(ego)
  latRef/1 -> Lateral Control/4(yRef), Sum1/1
  Bus Selector/4 -> Lateral Control/2(<r>), lat states/4  "<r>"
  Bus Selector/3 -> lat states/3, Bus Creator/4  "<psi>"
  Bus Selector/2 -> lat states/2  "<ydot>"
  Bus Selector/1 -> Sum1/2, Lateral Control/1(<Y>), lat states/1, Bus Creator/2  "<Y>"
  Mux1/1 -> Terminator/1
  Vehicle Body 3DOF Single Track/7 -> Mux1/6
  Vehicle Body 3DOF Single Track/6 -> Mux1/5
  Vehicle Body 3DOF Single Track/5 -> Mux1/4
  Vehicle Body 3DOF Single Track/2 -> Mux1/1
  Vehicle Body 3DOF Single Track/3 -> Mux1/2
  Vehicle Body 3DOF Single Track/4 -> Mux1/3
  Vehicle Body 3DOF Single Track/1 -> Bus Selector/1
  Gain/1 -> Vehicle Body 3DOF Single Track/3, Vehicle Body 3DOF Single Track/2
  Bus Selector/5 -> Bus Creator/1  "<X>"
  Bus Selector/6 -> Bus Creator/3  "<Xdot>"
  AND/1 -> Virtual Vehicle Following/4(extraSpaceFlag), On Delay/1, Regular Vehicle Following/4(extraSpaceFlag)  "extraSpaceFlag"
  Abs/1 -> vehWidth/2/1
  allVehicles/1 -> findLeader/2(all), virtualVehiclesManager/1(all)
  followerErrors/1(errors) -> safeErrors/1(errors)
  Regular Vehicle Following/3(gap) -> gap/1
  Regular Vehicle Following/1(u) -> controlChoice/2(follControl)
  Virtual Vehicle Following/1(u) -> Subsystem/1(u)
  Regular Vehicle Following/2(errors) -> Subsystem1/2(errors), errors/1
  Compare To Constant2/1 -> Lateral Control/3(startLaneChange)
  Lateral Control/1(delta) -> Vehicle Body 3DOF Single Track/1, Bus Creator/6
  maneuverState/1(state) -> system state/1, [state], Delay/1
  Virtual Vehicle Following/3(virtualGap) -> virtualGap/1
  [state] -> Compare To Constant2/1
  platoonState/1 -> Subsystem3/2(platoonStates), Subsystem2/3(platoonState)
  Subsystem2/1(longAdj) -> OR/1
  Delay/1 -> state/1  "u"
  strategy/1 -> Subsystem2/2(strategy), Subsystem3/1(strategy), virtualVehiclesManager/6(lcStrategy)
  Subsystem3/1(Out1) -> maneuverState/4(canStartLC)
  [state] -> findLeader/4(state)
  Virtual Vehicle Following/4(vLeaderInRange) -> controlChoice/5(vLeaderInRange)
  Triggered Subsystem/1(lcFlag) -> AND/2, findLeader/3(lcFlag), virtualVehiclesManager/3(lcFlag), Subsystem2/Enable

== system gg_plus_lc_platoon/Fd/Lateral Control ==
  <Y> : Inport
  <r> : Inport  Port=2
  startLaneChange : Inport  Port=3
  yRef : Inport  Port=4
  Demux2 : Demux
  Full State Observer : Subsystem
  Gain1 : Gain  Gain=Klat  Multiplication=Matrix(K*u)
  Integrator : Integrator  InitialCondition=y0
  Mux : Mux  Inputs=2
  Pad : dspsigops/Pad  padAlong=Columns  dimsToPad=1  valSrc=Specify via dialog  padVal=0  spec=Output size  padNumOutRowsSpecMethod=User-specified  numOutRows=4  padNumOutColsSpecMethod=User-specified  numOutCols=1  isVarDimsMode=off  padBeginning=0  padEnd=0  outSizeMode=User-specified  outSize=1  padSigAt=End  trunc_flag=None  roundingMode=Floor  overflowMode=off  truncOrWrapMode=Truncate  wrap_flag=None
      settings: SourceProductName=DSP System Toolbox  SourceProductBaseCode=DS
  Rate Limiter : RateLimiter  RisingSlewLimit=maxDeltaDot  FallingSlewLimit=-maxDeltaDot  SampleTimeMode=inherited
  Saturation : Saturate  UpperLimit=maxDelta  LowerLimit=-maxDelta
  Scope : Scope  NumInputPorts=4
  Scope1 : Scope
  Sum : Sum  Inputs=|+-
  Sum2 : Sum  Inputs=|+-
  Triggered Subsystem1 : Subsystem  TreatAsAtomicUnit=on
  delta : Outport
  wires:
  Rate Limiter/1 -> Full State Observer/2(delta), Scope1/1, delta/1  "delta"
  Demux2/1 -> Scope/1
  Integrator/1 -> Sum2/2, Pad/1
  Gain1/1 -> Saturation/1
  <r>/1 -> Mux/2
  Full State Observer/1(xhat) -> Sum/2, Demux2/1  "estStates"
  Sum/1 -> Gain1/1
  Pad/1 -> Sum/1
  Mux/1 -> Full State Observer/1(measuredOutputs)
  Demux2/4 -> Scope/4
  Demux2/2 -> Scope/2
  Sum2/1 -> Integrator/1
  Saturation/1 -> Rate Limiter/1
  Demux2/3 -> Scope/3
  Triggered Subsystem1/1(Out1) -> Sum2/1
  <Y>/1 -> Mux/1
  startLaneChange/1 -> Triggered Subsystem1/Trigger
  yRef/1 -> Triggered Subsystem1/1(In1)

== system gg_plus_lc_platoon/Fd/Regular Vehicle Following ==
  ego : Inport
  leader : Inport  Port=2
  leaderChange : Inport  Port=3
  extraSpaceFlag : Inport  Port=4
  Bus Selector : BusSelector  OutputSignals=X,Xdot,u
  Bus Selector1 : BusSelector  OutputSignals=X,Xdot
  Compare To Constant : simulink/Logic and Bit Operations/Compare To Constant  relop=<  const=5*maxHeadwayError  OutDataTypeStr=boolean
  Compute Errors : Subsystem
  Constant : Constant  Value=0
  Mux : Mux  Inputs=2
  Rate Limiter : RateLimiter  RisingSlewLimit=maxJerk  FallingSlewLimit=minJerk  SampleTimeMode=inherited
  Rate Limiter1 : RateLimiter  RisingSlewLimit=maxComfJerk  FallingSlewLimit=minComfJerk  SampleTimeMode=inherited
  Scope : Scope
  Scope2 : Scope
  Switch : Switch  Criteria=u2 > Threshold
  Switch1 : Switch  Criteria=u2 > Threshold
  Veh Following : Subsystem  TreatAsAtomicUnit=on
  Velocity Control : Subsystem  TreatAsAtomicUnit=on
  XOR : Logic  Operator=XOR  IconShape=distinctive  AllPortsSameDT=off  OutDataTypeStr=boolean
  comf saturation : Saturate  UpperLimit=maxComfAccel  LowerLimit=minComfAccel
  eh : Scope
  output : Scope
  safe saturation : Saturate  UpperLimit=maxAcceleration  LowerLimit=minAcceleration
  veh foll state : Scope  NumInputPorts=2
  u : Outport
  errors : Outport  Port=2
  gap : Outport  Port=3
  leaderInRange : Outport  Port=4
  wires:
  leaderChange/1 -> XOR/1
  Bus Selector/2 -> Velocity Control/1(velocity), Compute Errors/2(vf)  "<Xdot>"
  Bus Selector/1 -> Compute Errors/1(xf)  "<X>"
  Veh Following/1(u) -> Switch/1
  extraSpaceFlag/1 -> Compute Errors/5(extraSpaceFlag)
  Compute Errors/1(eh) -> eh/1, Compare To Constant/1, Scope/1, Veh Following/1(eh), Mux/1
  ego/1 -> Bus Selector/1
  Compute Errors/3("gap ") -> gap/1
  Compute Errors/4(unsafeFlag) -> Switch1/2, Scope2/1
  Rate Limiter1/1 -> Switch1/3  "sat(u)"
  Bus Selector/3 -> Veh Following/3(realInput), Velocity Control/2(realInput)  "<u>"
  Switch/1 -> safe saturation/1, veh foll state/2, comf saturation/1
  Switch1/1 -> u/1, output/1
  Rate Limiter/1 -> Switch1/1  "sat(u)"
  safe saturation/1 -> Rate Limiter/1
  comf saturation/1 -> Rate Limiter1/1
  Compute Errors/2(ev) -> Mux/2, Veh Following/2(ev)
  Velocity Control/1(u) -> Switch/3
  Bus Selector1/1 -> Compute Errors/3(xl)  "<X>"
  Mux/1 -> errors/1
  Compare To Constant/1 -> Switch/2, veh foll state/1, leaderInRange/1, XOR/2, Velocity Control/3(intReset)
  leader/1 -> Bus Selector1/1
  Bus Selector1/2 -> Compute Errors/4(vl)  "<Xdot>"
  XOR/1 -> Veh Following/4(intReset)
  Constant/1 -> Compute Errors/6(velFilterReset)

== system gg_plus_lc_platoon/Fd/Subsystem ==
  u : Inport
  state : Inport  Port=2
  Compare To Constant : simulink/Logic and Bit Operations/Compare To Constant  relop===  const=4  OutDataTypeStr=boolean
  Scope : Scope
  Switch1 : Switch  Criteria=u2 > Threshold
  comf saturation : Saturate  UpperLimit=maxComfAccel  LowerLimit=minComfAccel
  comf jerk : RateLimiter  RisingSlewLimit=maxComfJerk  FallingSlewLimit=minComfJerk  SampleTimeMode=inherited
  safe saturation : Saturate  UpperLimit=maxAcceleration  LowerLimit=minAcceleration
  safe jerk : RateLimiter  RisingSlewLimit=maxJerk  FallingSlewLimit=minJerk  SampleTimeMode=inherited
  sat(u) : Outport
  wires:
  Compare To Constant/1 -> Switch1/2
  Switch1/1 -> sat(u)/1, Scope/1
  comf jerk/1 -> Switch1/3
  u/1 -> safe saturation/1, comf saturation/1
  state/1 -> Compare To Constant/1
  comf saturation/1 -> comf jerk/1
  safe jerk/1 -> Switch1/1
  safe saturation/1 -> safe jerk/1

== system gg_plus_lc_platoon/Fd/Subsystem1 ==
  u : Inport
  errors : Inport  Port=2
  virtualErrors : Inport  Port=3
  extraSpaceFlag : Inport  Port=4
  AND1 : Logic  Inputs=4  IconShape=distinctive  AllPortsSameDT=off  OutDataTypeStr=boolean
  Memory : Memory
  Triggered Subsystem1 : Subsystem  TreatAsAtomicUnit=on
  safeErrors1 : Subsystem
  safeErrors2 : Subsystem
  steadyState : Subsystem
  longAdjDone : Outport
  wires:
  Memory/1 -> longAdjDone/1
  errors/1 -> safeErrors1/1(errors)
  Triggered Subsystem1/1(Out1) -> Memory/1
  AND1/1 -> Triggered Subsystem1/Trigger
  safeErrors2/1(safetyFlag) -> AND1/3
  virtualErrors/1 -> safeErrors2/1(errors)
  extraSpaceFlag/1 -> AND1/4
  steadyState/1(ssFlag) -> AND1/1
  safeErrors1/1(safetyFlag) -> AND1/2
  u/1 -> steadyState/1(u)

== system gg_plus_lc_platoon/Fd/Subsystem2 ==
  posInPlatoon : Inport
  strategy : Inport  Port=2
  platoonState : Inport  Port=3
  Enable : EnablePort
  MATLAB Function : MATLAB Function  TreatAsAtomicUnit=on
  longAdj : Outport
  wires:
  strategy/1 -> MATLAB Function/1(strategy)
  posInPlatoon/1 -> MATLAB Function/2(posInPlatoon)
  platoonState/1 -> MATLAB Function/3(platoonState)
  MATLAB Function/1(longAdjFlag) -> longAdj/1

== system gg_plus_lc_platoon/Fd/Subsystem3 ==
  strategy : Inport
  platoonStates : Inport  Port=2
  Compare To Constant : simulink/Logic and Bit Operations/Compare To Constant  relop=>  const=1  OutDataTypeStr=boolean
  Compare To Constant1 : simulink/Logic and Bit Operations/Compare To Constant  relop=>  const=2  OutDataTypeStr=boolean
  OR : Logic  Operator=OR  IconShape=distinctive  AllPortsSameDT=off  OutDataTypeStr=boolean
  Selector : Selector  IndexOptions=Index vector (port)  Indices=[1 3]  OutputSizes=1
  Width : Width
  Out1 : Outport
  wires:
  strategy/1 -> Compare To Constant/1
  Compare To Constant/1 -> OR/1
  OR/1 -> Out1/1
  platoonStates/1 -> Width/1, Selector/1
  Width/1 -> Selector/2
  Selector/1 -> Compare To Constant1/1
  Compare To Constant1/1 -> OR/2

== system gg_plus_lc_platoon/Fd/Triggered Subsystem ==
  Trigger : TriggerPort  VariantControl=Variant
  Constant : Constant
  lcFlag : Outport  InitialOutput=0
  wires:
  Constant/1 -> lcFlag/1
